simulink model "sl_subsys_fcncallerr8"  (Simulink 7.6)
settings: Solver=FixedStepDiscrete  StartTime=0.0  StopTime=10.0  FixedStep=1  RelTol=1e-3
Description:
  | Function-call subsystem cycle data dependency violation
  | 
  | To execute f2() we require that its data source, f1(),
  | execute before its initiator, chart2, so that sig1 is
  | valid. Likewise, to execute f1() we require that its data
  | source, f2(), execute before its initiator, chart1, so that
  | sig2 is valid. Hence the data dependency violation.
settings Model: Creator=The MathWorks Inc.  CovMetricSettings=d  ExtModeAutoUpdateStatusClock=off
settings OptimizationCC: BlockReduction=off  BooleanDataType=off  InlineInvariantSignals=on  InitFltsAndDblsToZero=on
settings DebuggingCC: SaveWithParameterizedLinksMsg=none  SignalResolutionControl=TryResolveAllWithWarning  SolverPrmCheckMsg=none  MultiTaskDSMMsg=warning  MultiTaskCondExecSysMsg=none  UnconnectedInputMsg=none  UnconnectedOutputMsg=none  UnconnectedLineMsg=none
settings HardwareCC: TargetUnknown=on
settings SFSimCC: SimParseCustomCode=off
settings RTWCC: IncludeERTFirstTime=on
settings CodeAppCC: CustomSymbolStrFcn=$F$N$M
settings GRTTargetCC: TargetFcnLib=ansi_tfl_tmw.mat

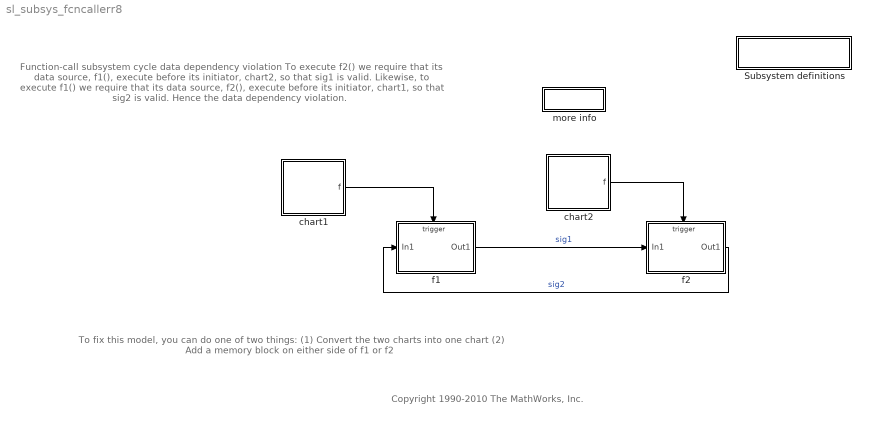
== system sl_subsys_fcncallerr8 ==
  note: To fix this model, you can do one of two things:
      | (1) Convert the two charts into one chart
      | (2) Add a memory block on either side of f1 or f2
  note: Function-call subsystem cycle data dependency violation
      |
      | To execute f2() we require that its data source, f1(),
      | execute before its initiator, chart2, so that sig1 is
      | valid. Likewise, to execute f1() we require that its data
      | source, f2(), execute before its initiator, chart1, so that
      | sig2 is valid. Hence the data dependency violation.
  note: Copyright 1990-2010 The MathWorks, Inc.
  " Subsystem definitions" : Subsystem
      settings: OpenFcn=helpview([matlabroot,'/toolbox/simulink/simdemos/simfeatures/html/sl_subsys_definitions.html']);
      mask Display: disp('Subsystem\ndefinitions')
  chart1 : Stateflow chart  TreatAsAtomicUnit=on
  chart2 : Stateflow chart  TreatAsAtomicUnit=on
  f1 : Subsystem  TreatAsAtomicUnit=on
  f2 : Subsystem  TreatAsAtomicUnit=on
  more info : Subsystem
      mask Display: disp(get_param(gcb,'name'))
  wires:
  chart1/1(f) -> f1/Trigger
  chart2/1(f) -> f2/Trigger
  f1/1(Out1) -> f2/1(In1)  "sig1"
  f2/1(Out1) -> f1/1(In1)  "sig2"

== system sl_subsys_fcncallerr8/ Subsystem definitions ==

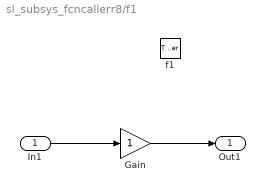
== system sl_subsys_fcncallerr8/f1 ==
  In1 : Inport
  f1 : TriggerPort  TriggerType=function-call
  Gain : Gain  SaturateOnIntegerOverflow=on  OutDataTypeStr=Inherit: Same as input  ParamDataTypeStr=Inherit: Same as input
  Out1 : Outport
  wires:
  In1/1 -> Gain/1
  Gain/1 -> Out1/1

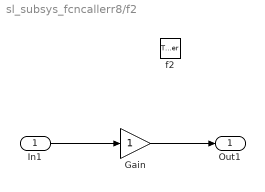
== system sl_subsys_fcncallerr8/f2 ==
  In1 : Inport
  f2 : TriggerPort  TriggerType=function-call
  Gain : Gain  SaturateOnIntegerOverflow=on  OutDataTypeStr=Inherit: Same as input  ParamDataTypeStr=Inherit: Same as input
  Out1 : Outport
  wires:
  In1/1 -> Gain/1
  Gain/1 -> Out1/1

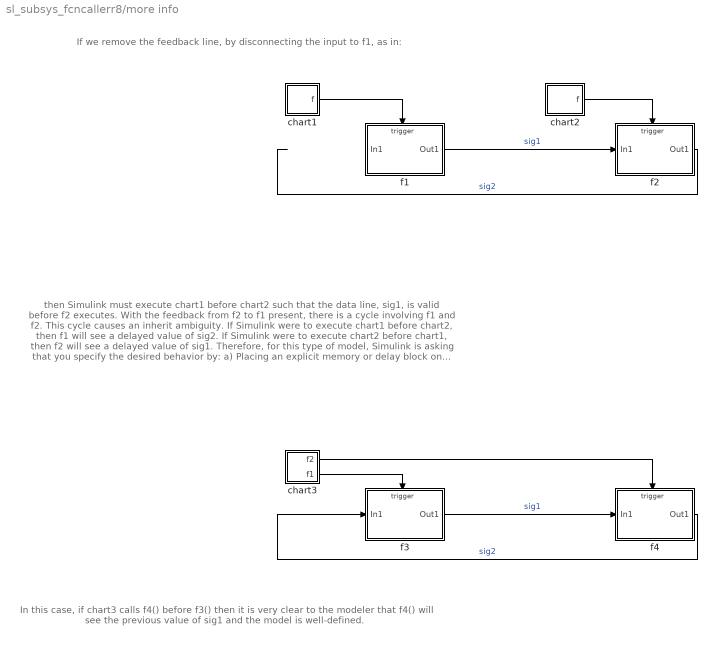
== system sl_subsys_fcncallerr8/more info ==
  note: If we remove the feedback line, by disconnecting the input to f1, as in:
  note: then Simulink must execute chart1 before chart2 such that the data
      | line, sig1, is valid before f2 executes. With the feedback from
      | f2 to f1 present, there is a cycle involving f1 and f2.  This cycle
      | causes an inherit ambiguity. If Simulink were to execute chart1
      | before chart2, then f1 will see a delayed value of sig2. If
      | Simulink were to execute chart2 before chart1, then f2 will see a
      | delayed value of sig1.
      |
      | Therefore, for this type of model, Simulink is asking that you
      | specify the desired behavior by:
      |
      |   a) Placing an explicit memory or delay block on either sig1 or sig2
      |      such that the delay is clearly spelled out.
      |   b) Updating the model to have a single initiator as in:
  note: In this case, if chart3 calls f4() before f3() then it is very
      |      clear to the modeler that f4() will see the previous value of sig1 and
      |      the model is well-defined.
  chart1 : Stateflow chart  TreatAsAtomicUnit=on
  chart2 : Stateflow chart  TreatAsAtomicUnit=on
  chart3 : Stateflow chart  TreatAsAtomicUnit=on
  f1 : Subsystem  TreatAsAtomicUnit=on
  f2 : Subsystem  TreatAsAtomicUnit=on
  f3 : Subsystem  TreatAsAtomicUnit=on
  f4 : Subsystem  TreatAsAtomicUnit=on
  wires:
  chart1/1(f) -> f1/Trigger
  chart2/1(f) -> f2/Trigger
  f1/1(Out1) -> f2/1(In1)  "sig1"
  f2/1(Out1) -> ?  "sig2"
  chart3/1(f2) -> f4/Trigger
  f3/1(Out1) -> f4/1(In1)  "sig1"
  f4/1(Out1) -> f3/1(In1)  "sig2"
  chart3/2(f1) -> f3/Trigger

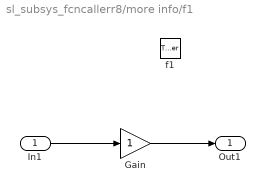
== system sl_subsys_fcncallerr8/more info/f1 ==
  In1 : Inport
  f1 : TriggerPort  TriggerType=function-call
  Gain : Gain  SaturateOnIntegerOverflow=on  OutDataTypeStr=Inherit: Same as input  ParamDataTypeStr=Inherit: Same as input
  Out1 : Outport
  wires:
  Gain/1 -> Out1/1
  In1/1 -> Gain/1

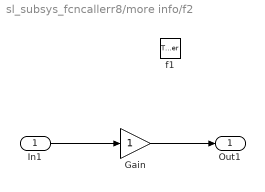
== system sl_subsys_fcncallerr8/more info/f2 ==
  In1 : Inport
  f1 : TriggerPort  TriggerType=function-call
  Gain : Gain  SaturateOnIntegerOverflow=on  OutDataTypeStr=Inherit: Same as input  ParamDataTypeStr=Inherit: Same as input
  Out1 : Outport
  wires:
  Gain/1 -> Out1/1
  In1/1 -> Gain/1

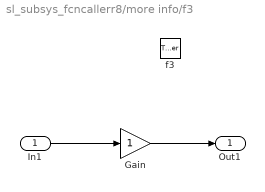
== system sl_subsys_fcncallerr8/more info/f3 ==
  In1 : Inport
  f3 : TriggerPort  TriggerType=function-call
  Gain : Gain  SaturateOnIntegerOverflow=on  OutDataTypeStr=Inherit: Same as input  ParamDataTypeStr=Inherit: Same as input
  Out1 : Outport
  wires:
  In1/1 -> Gain/1
  Gain/1 -> Out1/1

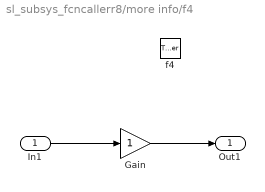
== system sl_subsys_fcncallerr8/more info/f4 ==
  In1 : Inport
  f4 : TriggerPort  TriggerType=function-call
  Gain : Gain  SaturateOnIntegerOverflow=on  OutDataTypeStr=Inherit: Same as input  ParamDataTypeStr=Inherit: Same as input
  Out1 : Outport
  wires:
  In1/1 -> Gain/1
  Gain/1 -> Out1/1

== stateflow chart chart2 ==
  state one/
    entry: f;
  state two/
    entry: f;
  one -> two
  two -> one
  (default) -> one
  events: f output FUNCTION_CALL_EVENT

== stateflow chart chart1 ==
  state one/
    entry: f;
  state two/
    entry: f;
  one -> two
  two -> one
  (default) -> one
  events: f output FUNCTION_CALL_EVENT

== stateflow chart more info/chart1 ==
  state one/
    entry: f;
  state two/
    entry: f;
  one -> two
  two -> one
  (default) -> one
  events: f output FUNCTION_CALL_EVENT

== stateflow chart more info/chart2 ==
  state one/
    entry: f;
  state two/
    entry: f;
  one -> two
  two -> one
  (default) -> one
  events: f output FUNCTION_CALL_EVENT

== stateflow chart more info/chart3 ==
  state one/
    entry: f1;f2;
  state two/
    entry: f2;f1;
  one -> two
  two -> one
  (default) -> one
  events: f2 output FUNCTION_CALL_EVENT; f1 output FUNCTION_CALL_EVENT
